simulink model "PI"  (Simulink 7.9)
settings: Solver=ode45  StartTime=0.0  StopTime=3  RelTol=1e-3
settings Model: Creator=Lithium  LastModifiedBy=Lithium
settings DebuggingCC: FcnCallInpInsideContextMsg=Use local settings
settings GRTTargetCC: CombineOutputUpdateFcns=off  GRTInterface=on

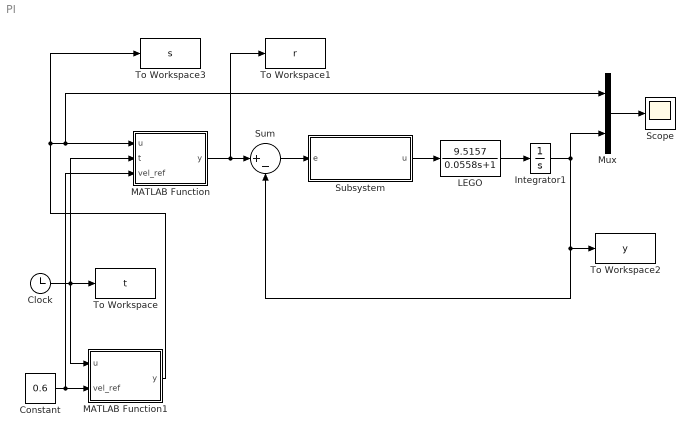
== system PI ==
  Clock : Clock
  Constant : Constant  Value=0.6
  Integrator1 : Integrator
  LEGO : TransferFcn  Numerator=[9.5157]  Denominator=[0.0558 1]
  MATLAB Function : MATLAB Function  TreatAsAtomicUnit=on
  MATLAB Function1 : MATLAB Function  TreatAsAtomicUnit=on
  Mux : Mux  Inputs=2
  Scope : Scope
  Subsystem : Subsystem
  Sum : Sum  Inputs=|+-
  To Workspace : ToWorkspace  VariableName=t  SampleTime=-1
  To Workspace1 : ToWorkspace  VariableName=r  SampleTime=-1
  To Workspace2 : ToWorkspace  VariableName=y  SampleTime=-1
  To Workspace3 : ToWorkspace  VariableName=s  SampleTime=-1
  wires:
  Mux/1 -> Scope/1
  LEGO/1 -> Integrator1/1
  Integrator1/1 -> Mux/2, Sum/2, To Workspace2/1
  Subsystem/1(u) -> LEGO/1
  Sum/1 -> Subsystem/1(e)
  Clock/1 -> To Workspace/1, MATLAB Function/2(t), MATLAB Function1/1(u)
  MATLAB Function/1(y) -> Sum/1, To Workspace1/1
  MATLAB Function1/1(y) -> Mux/1, MATLAB Function/1(u), To Workspace3/1
  Constant/1 -> MATLAB Function1/2(vel_ref), MATLAB Function/3(vel_ref)

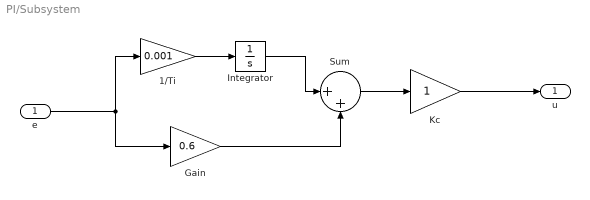
== system PI/Subsystem ==
  e : Inport
  1/Ti : Gain  Gain=0.001
  Gain : Gain  Gain=0.6
  Integrator : Integrator
  Kc : Gain
  Sum : Sum  Inputs=|++
  u : Outport
  wires:
  Integrator/1 -> Sum/1
  Gain/1 -> Sum/2
  e/1 -> 1/Ti/1, Gain/1
  1/Ti/1 -> Integrator/1
  Sum/1 -> Kc/1
  Kc/1 -> u/1

== matlab function MATLAB Function1 ==
  data: u input double; y output double; vel_ref input double
function y= fcn(u, vel_ref)
%#codegen

Wmax = vel_ref;


if(u <= 0.5)
    y = Wmax;
else
    y = 0;
end

== matlab function MATLAB Function ==
  data: u input double; y output double; t input double; vel_ref input double
function y = fcn(u, t, vel_ref)
%#codegen

Wmax = u;
thao = 0.005;

if (Wmax > 0)
 
   if((vel_ref/0.7)*t <= Wmax) 
          y = (vel_ref/0.7)*t;
      else
          y = Wmax;
   end
else
    
    y = (vel_ref*(t^2)/0.7) + (((0.7*vel_ref)/2) - (vel_ref/1.4)*(0.7-t)^2);


end
